simulink model "Car_Trailer_SimuLinkModel"  (R2022b)
settings: Solver=VariableStepAuto  StartTime=0.0  StopTime=10.0  RelTol=1e-3
settings Model: Creator=vidus  LastModifiedBy=vidus

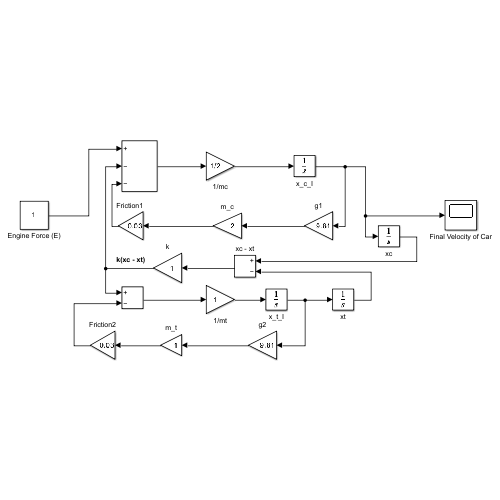
[thumbnail: Simulink's stored preview of the top-level diagram]
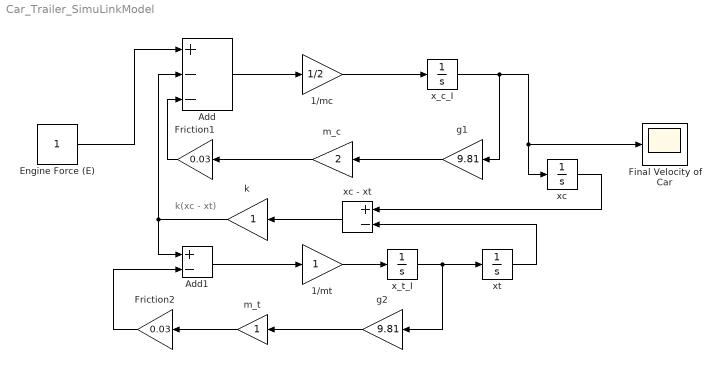
== system Car_Trailer_SimuLinkModel ==
  note: k(xc - xt)
  1/mc : Gain  Gain=1/2
  1/mt : Gain
  Add : Sum  Inputs=+--
  Add1 : Sum  Inputs=+-
  Engine Force (E) : Constant
  Final Velocity of Car : Scope
  "Friction1 " : Gain  Gain=0.03
  Friction2 : Gain  Gain=0.03
  g1 : Gain  Gain=9.81
  g2 : Gain  Gain=9.81
  k : Gain
  m_c : Gain  Gain=2
  m_t : Gain
  x_c_I : Integrator
  x_t_I : Integrator
  xc : Integrator
  xc - xt : Sum  Inputs=+-
  xt : Integrator
  wires:
  Friction2/1 -> Add1/2
  1/mt/1 -> x_t_I/1
  m_t/1 -> Friction2/1
  xc - xt/1 -> k/1
  1/mc/1 -> x_c_I/1
  k/1 -> Add/2, Add1/1
  Add1/1 -> 1/mt/1
  m_c/1 -> "Friction1 "/1
  "Friction1 "/1 -> Add/3
  Engine Force (E)/1 -> Add/1
  xc/1 -> xc - xt/1
  g2/1 -> m_t/1
  x_c_I/1 -> g1/1, Final Velocity of Car/1, xc/1
  Add/1 -> 1/mc/1
  xt/1 -> xc - xt/2
  x_t_I/1 -> g2/1, xt/1
  g1/1 -> m_c/1
